simulink model "Traffic_Light_2021b"  (R2021b)
settings: Solver=FixedStepDiscrete  StartTime=0.0  StopTime=50  FixedStep=1e-3  RelTol=1e-3  EnableMultiTasking=on
libraries: arduinolib x3
settings Model: NumberOfSteps=5000  ExtModeTrigDuration=2  Creator=gaafa  LastModifiedBy=gaafa
settings OptimizationCC: EnhancedBackFolding=on  PassReuseOutputArgsAs=Individual arguments  ZeroExternalMemoryAtStartup=off  ZeroInternalMemoryAtStartup=off  MaxStackSize=64  OptimizeBlockOrder=speed  DifferentSizesBufferReuse=on  OptimizationCustomize=off  EfficientTunableParamExpr=on
settings DebuggingCC: ParameterTunabilityLossMsg=error  UnconnectedInputMsg=none  UnconnectedOutputMsg=none  UnconnectedLineMsg=none
settings HardwareCC: ProdBitPerInt=16  ProdBitPerPointer=16  ProdBitPerSizeT=16  ProdBitPerPtrDiffT=16  ProdLargestAtomicFloat=None  ProdWordSize=8  ProdHWDeviceType=Atmel->AVR
settings ModelReferenceCC: EnableRefExpFcnMdlSchedulingChecks=off
settings SFSimCC: MATLABDynamicMemAlloc=off
settings RTWCC: Description=Embedded Coder  SystemTargetFile=ert.tlc  HardwareBoard=Arduino Uno  TemplateMakefile=ert_default_tmf  Toolchain=Arduino AVR  BuildConfiguration=Faster Runs  DLArmComputeVersion=20.02.1
settings CodeAppCC: ForceParamTrailComments=on  IgnoreCustomStorageClasses=off  OperatorAnnotations=on  SimulinkDataObjDesc=on  SFDataObjDesc=on  InsertBlockDesc=on
settings ERTTargetCC: SupportContinuousTime=on  SupportVariableSizeSignals=on  ExtModeTransport=3  ExtModeStaticAlloc=on  ExtModeStaticAllocSize=250  ExtModeMexFile=ext_xcp  ExtModeIntrfLevel=Level2 - Open

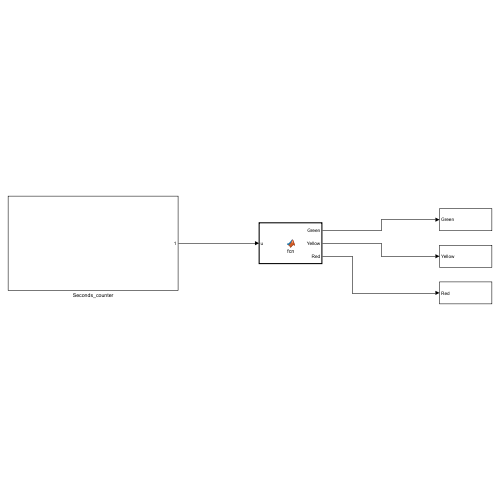
[thumbnail: Simulink's stored preview of the top-level diagram]
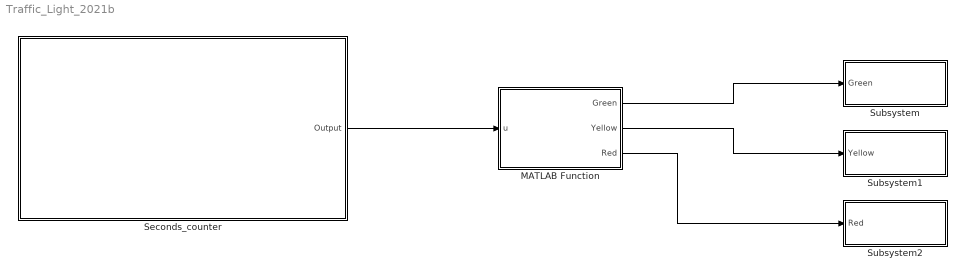
== system Traffic_Light_2021b ==
  MATLAB Function : MATLAB Function  TreatAsAtomicUnit=on
  Seconds_counter : Subsystem
  Subsystem : Subsystem
  Subsystem1 : Subsystem
  Subsystem2 : Subsystem
  wires:
  Seconds_counter/1(Output) -> MATLAB Function/1(u)
  MATLAB Function/1(Green) -> Subsystem/1(Green)
  MATLAB Function/2(Yellow) -> Subsystem1/1(Yellow)
  MATLAB Function/3(Red) -> Subsystem2/1(Red)

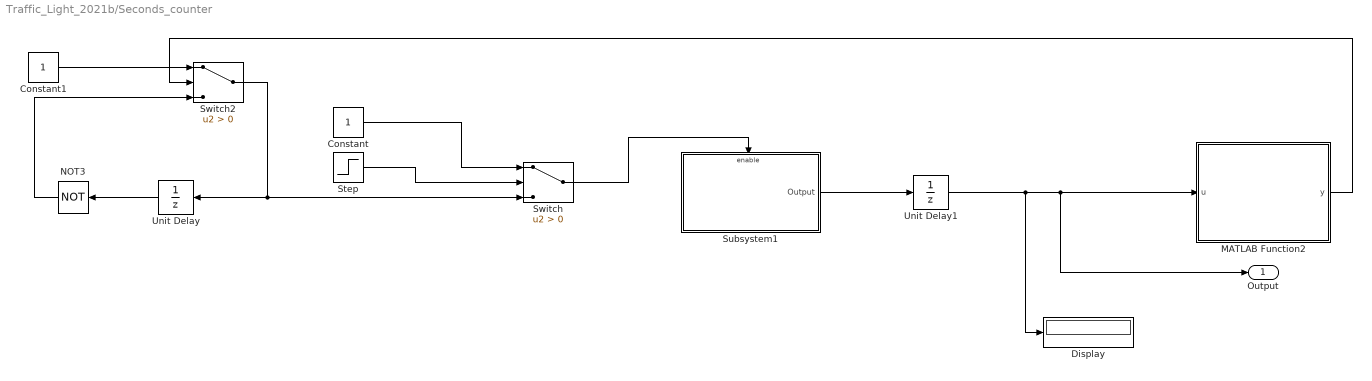
== system Traffic_Light_2021b/Seconds_counter ==
  Constant : Constant
  Constant1 : Constant
  Display : Display
  MATLAB Function2 : MATLAB Function  TreatAsAtomicUnit=on
  NOT3 : Logic  Operator=NOT  IconShape=distinctive  AllPortsSameDT=off  OutDataTypeStr=boolean
  Step : Step  Time=2  Before=1  After=0  SampleTime=1
  Subsystem1 : Subsystem
  Switch : Switch  Criteria=u2 > Threshold
  Switch2 : Switch  Criteria=u2 > Threshold
  Unit Delay : UnitDelay  SampleTime=-1  HasFrameUpgradeWarning=on
  Unit Delay1 : UnitDelay  InitialCondition=1  SampleTime=-1  HasFrameUpgradeWarning=on
  Output : Outport
  wires:
  Constant1/1 -> Switch2/1
  NOT3/1 -> Switch2/3
  Switch2/1 -> Unit Delay/1, Switch/3
  Step/1 -> Switch/2
  Constant/1 -> Switch/1
  Subsystem1/1(Output) -> Unit Delay1/1
  Unit Delay/1 -> NOT3/1
  MATLAB Function2/1(y) -> Switch2/2
  Unit Delay1/1 -> Display/1, Output/1, MATLAB Function2/1(u)
  Switch/1 -> Subsystem1/Enable

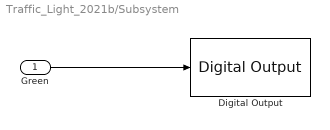
== system Traffic_Light_2021b/Subsystem ==
  Green : Inport
  Digital Output : arduinolib/Digital Output  pinNumber=2  Direction=output  blockPlatform=arduino
  wires:
  Green/1 -> Digital Output/1

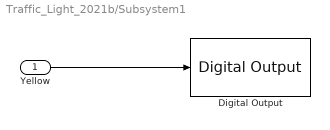
== system Traffic_Light_2021b/Subsystem1 ==
  Yellow : Inport
  Digital Output : arduinolib/Digital Output  pinNumber=3  Direction=output  blockPlatform=arduino
  wires:
  Yellow/1 -> Digital Output/1

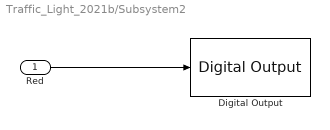
== system Traffic_Light_2021b/Subsystem2 ==
  Red : Inport
  Digital Output : arduinolib/Digital Output  pinNumber=4  Direction=output  blockPlatform=arduino
  wires:
  Red/1 -> Digital Output/1

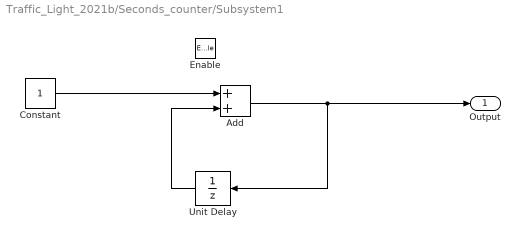
== system Traffic_Light_2021b/Seconds_counter/Subsystem1 ==
  Enable : EnablePort  StatesWhenEnabling=reset
  Add : Sum
  Constant : Constant
  Unit Delay : UnitDelay  InitialCondition=1  HasFrameUpgradeWarning=on
  Output : Outport
  wires:
  Add/1 -> Unit Delay/1, Output/1
  Unit Delay/1 -> Add/2
  Constant/1 -> Add/1

== matlab function Traffic_Light_2021b/Seconds_counter/MATLAB Function2 ==
  data: u input; y output
function y = Seconds_Detector(u)
y=1;
if (u == 29)
    y=0;
end

== matlab function Traffic_Light_2021b/MATLAB Function ==
  data: u input; Green output; Yellow output; Red output
function [Green , Yellow , Red ] = fcn(u)
Green = 0 ;
Yellow = 0 ; 
Red  = 0;

if ( u >=0 && u <=15 )
    Green = 1;
elseif (u >=15 && u <=20)
    Yellow = 1 ;
elseif (u >=20 && u <=30)
    Red  = 1;
end
